simulink model "Distribute4_Model"  (R2024b)
settings: Solver=VariableStepAuto  StartTime=0.0  StopTime=10.0  RelTol=1e-3
libraries: NSA_DEVS_SINKS x6, NSA_DEVS_LOGISTICS x4, NSA_DEVS_SOURCES x2, NSA_DEVS_ROUTING x1
settings Model: Creator=david  LastModifiedBy=peter
settings RTWCC: GPUComputeCapability=3.5

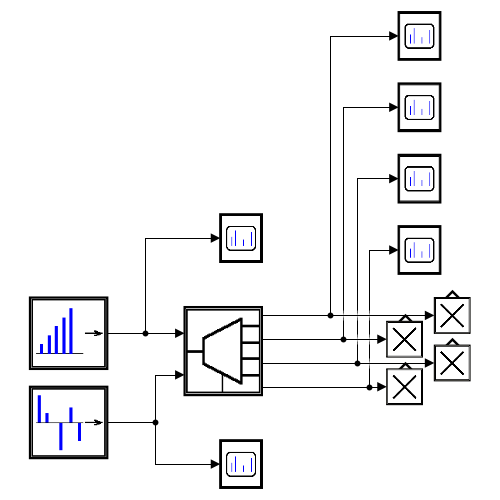
[thumbnail: Simulink's stored preview of the top-level diagram]
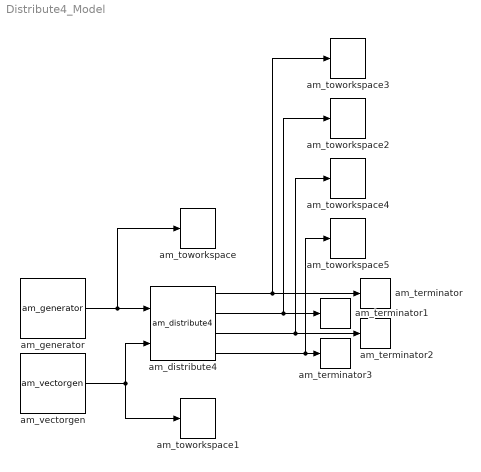
== system Distribute4_Model ==
  am_distribute4 : NSA_DEVS_ROUTING/am_distribute4  port0=1  field="\"\""  tau=[0,1]  debug=0
      settings: SourceProductName=Routing
  am_generator : NSA_DEVS_SOURCES/am_generator  tG=1  n0=1  nG=100  tD=[0,2]  debug=0
      settings: SourceProductName=Sources
  am_terminator{,1..3} (4 alike) : NSA_DEVS_LOGISTICS/am_terminator  tau=[0,1]  debug=0
      settings: SourceProductName=Logistics
  am_toworkspace : NSA_DEVS_SINKS/am_toworkspace  varname="\"genOut\""  t0=0  format="\"vector\""  tau=[0,5]  debug=0
      settings: SourceProductName=Sinks
  am_toworkspace1 : NSA_DEVS_SINKS/am_toworkspace  varname="\"vgenOut\""  t0=0  format="\"vector\""  tau=[0,5]  debug=0
      settings: SourceProductName=Sinks
  am_toworkspace2 : NSA_DEVS_SINKS/am_toworkspace  varname="\"dist2Out\""  t0=0  format="\"vector\""  tau=[0,5]  debug=0
      settings: SourceProductName=Sinks
  am_toworkspace3 : NSA_DEVS_SINKS/am_toworkspace  varname="\"dist1Out\""  t0=0  format="\"vector\""  tau=[0,5]  debug=0
      settings: SourceProductName=Sinks
  am_toworkspace4 : NSA_DEVS_SINKS/am_toworkspace  varname="\"dist3Out\""  t0=0  format="\"vector\""  tau=[0,5]  debug=0
      settings: SourceProductName=Sinks
  am_toworkspace5 : NSA_DEVS_SINKS/am_toworkspace  varname="\"dist4Out\""  t0=0  format="\"vector\""  tau=[0,5]  debug=0
      settings: SourceProductName=Sinks
  am_vectorgen : NSA_DEVS_SOURCES/am_vectorgen  tvec=[1.5 2.5 4.5 6.5 8.5 10.5]  yvec=[2, 3, 2, 1, 4, 1]  tau=[0,1]  debug=0
      settings: SourceProductName=Sources
  wires:
  am_generator/1 -> am_distribute4/1, am_toworkspace/1
  am_distribute4/1 -> am_terminator/1, am_toworkspace3/1
  am_distribute4/2 -> am_terminator1/1, am_toworkspace2/1
  am_distribute4/3 -> am_terminator2/1, am_toworkspace4/1
  am_vectorgen/1 -> am_distribute4/2, am_toworkspace1/1
  am_distribute4/4 -> am_toworkspace5/1, am_terminator3/1
